simulink model "course_loop"  (Simulink 9.0)
settings: Solver=VariableStepAuto  StartTime=0.0  StopTime=30  RelTol=1e-3
InitFcn:
  | param_chap6
values from neighbouring files (symbols this model uses):
  G = getGains(P,G)    [param_chap6.m]
libraries: cstblocks x2, simulink x1
settings Model: SuppressorTable=22 serialization::archive 11 0 6 0 0 0 0 0  Creator=leonardopedroso  LastModifiedBy=leonardopedroso
settings DataIOCC: SaveFormat=Dataset
settings OptimizationCC: LifeSpan=auto
settings DebuggingCC: UnderspecifiedInitializationDetection=Simplified  MergeDetectMultiDrivingBlocksExec=error  SFUnexpectedBacktrackingDiag=error  SFNoUnconditionalDefaultTransitionDiag=error  SFExecutionAtInitializationDiag=warning
settings HardwareCC: ProdBitPerPointer=64  ProdBitPerSizeT=64  ProdBitPerPtrDiffT=64  ProdLargestAtomicFloat=Float  ProdIntDivRoundTo=Zero  ProdEndianess=LittleEndian  ProdWordSize=64  ProdHWDeviceType=Intel->x86-64 (Windows64)
settings ModelReferenceCC: PropagateSignalLabelsOutOfModel=on
settings CodeAppCC: StateflowObjectComments=off
settings GRTTargetCC: TargetLangStandard=C99 (ISO)
settings ConfigComp: CovMetricSettings=dwe  CovHtmlReporting=off  CovSaveCumulativeToWorkspaceVar=off  CovSaveSingleToWorkspaceVar=off  CovExternalEMLEnable=on

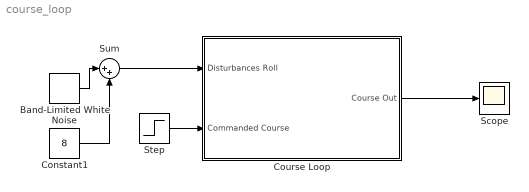
== system course_loop ==
  Band-Limited White Noise : simulink/Sources/Band-Limited White Noise  Cov=[0.1]  Ts=0.1  seed=[23341]
  Constant1 : Constant  Value=8
  Course Loop : Subsystem
  Scope : Scope
  Step : Step  After=pi/6  SampleTime=0
  Sum : Sum  Inputs=|++
  wires:
  Step/1 -> Course Loop/2(Commanded Course)
  Course Loop/1("Course Out ") -> Scope/1
  Band-Limited White Noise/1 -> Sum/1
  Constant1/1 -> Sum/2
  Sum/1 -> Course Loop/1(Disturbances Roll)

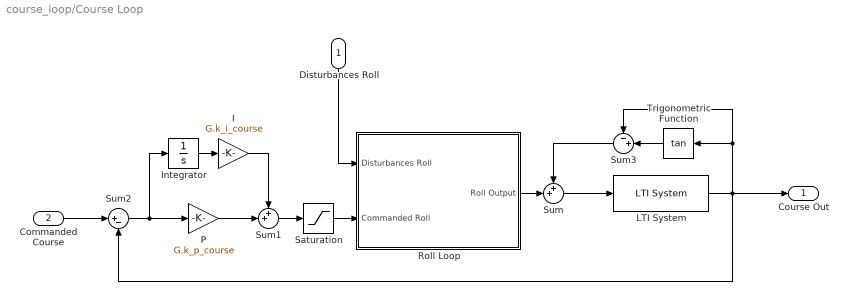
== system course_loop/Course Loop ==
  Disturbances Roll : Inport
  Commanded Course : Inport  Port=2
  I : Gain  Gain=G.k_i_course
  Integrator : Integrator
  LTI System : cstblocks/LTI System  sys=T_chi_phi  IC=[]
  P : Gain  Gain=G.k_p_course
  "Roll Loop " : Subsystem
  Saturation : Saturate  UpperLimit=pi/6  LowerLimit=-pi/6
  Sum : Sum  Inputs=++|
  Sum1 : Sum  Inputs=++|
  Sum2 : Sum  Inputs=|+-
  Sum3 : Sum  Inputs=-+|
  Trigonometric Function : Trigonometry  Operator=tan
  "Course Out " : Outport
  wires:
  "Roll Loop "/1(Roll Output) -> Sum/2
  P/1 -> Sum1/2
  Integrator/1 -> I/1
  LTI System/1 -> Sum2/2, Sum3/1, Trigonometric Function/1, "Course Out "/1
  Disturbances Roll/1 -> "Roll Loop "/1("Disturbances Roll ")
  Sum/1 -> LTI System/1
  I/1 -> Sum1/1
  Sum2/1 -> Integrator/1, P/1
  Commanded Course/1 -> Sum2/1
  Sum3/1 -> Sum/1
  Trigonometric Function/1 -> Sum3/2
  Sum1/1 -> Saturation/1
  Saturation/1 -> "Roll Loop "/2(Commanded Roll)

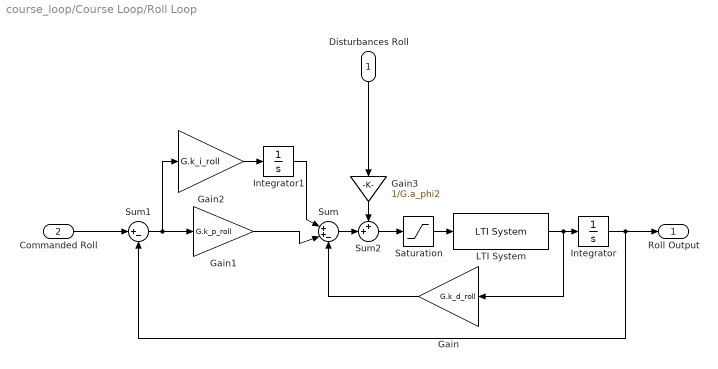
== system course_loop/Course Loop/Roll Loop  ==
  "Disturbances Roll " : Inport
  Commanded Roll : Inport  Port=2
  Gain : Gain  Gain=G.k_d_roll
  Gain1 : Gain  Gain=G.k_p_roll
  Gain2 : Gain  Gain=G.k_i_roll
  Gain3 : Gain  Gain=1/G.a_phi2
  Integrator : Integrator
  Integrator1 : Integrator
  LTI System : cstblocks/LTI System  sys=T_p_delta_a  IC=[]
  Saturation : Saturate  UpperLimit=G.delta_a_max  LowerLimit=-G.delta_a_max
  Sum : Sum  Inputs=|++-
  Sum1 : Sum  Inputs=|+-
  Sum2 : Sum  Inputs=++|
  Roll Output : Outport
  wires:
  Integrator/1 -> Roll Output/1, Sum1/2
  Gain1/1 -> Sum/2
  Gain/1 -> Sum/3
  Sum1/1 -> Gain2/1, Gain1/1
  Gain2/1 -> Integrator1/1
  Integrator1/1 -> Sum/1
  Commanded Roll/1 -> Sum1/1
  Sum/1 -> Sum2/2
  Gain3/1 -> Sum2/1
  "Disturbances Roll "/1 -> Gain3/1
  Sum2/1 -> Saturation/1
  Saturation/1 -> LTI System/1
  LTI System/1 -> Integrator/1, Gain/1
